simulink model "exjobbtest"  (R2019b)
settings: Solver=VariableStepAuto  StartTime=0.0  StopTime=50  RelTol=1e-3
libraries: simulink x1
settings Model: Creator=Jonathan  LastModifiedBy=Jonathan

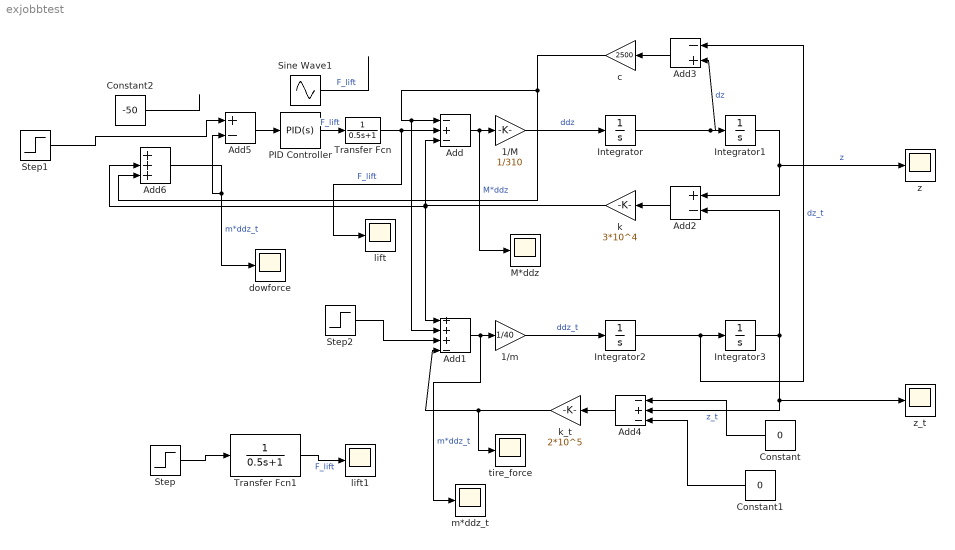
== system exjobbtest ==
  1/M : Gain  Gain=1/310
  1/m : Gain  Gain=1/40
  Add : Sum  Inputs=-+-
  Add1 : Sum  Inputs=+++-
  Add2 : Sum  Inputs=+-
  Add3 : Sum  Inputs=-+
  Add4 : Sum  Inputs=-+-
  Add5 : Sum  Inputs=+-
  Add6 : Sum  Inputs=+++
  Constant : Constant  Value=0
  Constant1 : Constant  Value=0
  Constant2 : Constant  Value=-50
  Integrator{,1..3} (4 alike) : Integrator
  M*ddz : Scope
  PID Controller : simulink/Continuous/PID Controller  Controller=PID  Form=Parallel  TimeDomain=Continuous-time  SampleTime=-1  IntegratorMethod=Forward Euler  FilterMethod=Forward Euler  ControllerParametersSource=internal  P=2.01508415148749  I=5.2932455765264  D=0.107676249350259  UseFilter=on  N=622.23893697959  TunerSelectOption=Transfer Function Based (PID Tuner App)  InitialConditionSource=internal  InitialConditionForIntegrator=0  InitialConditionForFilter=0  DifferentiatorICPrevScaledInput=0  ExternalReset=none  TrackingMode=off  Kt=1  LimitOutput=off  UpperSaturationLimit=inf  LowerSaturationLimit=-inf  LinearizeAsGain=on  AntiWindupMode=none  Kb=1  POutMin=[]  POutMax=[]  IOutMin=[]  IOutMax=[]  DOutMin=[]  DOutMax=[]  NOutMin=[]  NOutMax=[]  SumOutMin=[]  SumOutMax=[]  SaturationOutMin=[]  SaturationOutMax=[]  PParamMin=[]  PParamMax=[]  IParamMin=[]  IParamMax=[]  DParamMin=[]  DParamMax=[]  NParamMin=[]  NParamMax=[]  KbParamMin=[]  KbParamMax=[]  KtParamMin=[]  KtParamMax=[]  KbOutMin=[]  KbOutMax=[]  KtOutMin=[]  KtOutMax=[]  IntegratorOutMin=[]  IntegratorOutMax=[]  FilterOutMin=[]  FilterOutMax=[]  SumI1OutMin=[]  SumI1OutMax=[]  SumI2OutMin=[]  SumI2OutMax=[]  SumI3OutMin=[]  SumI3OutMax=[]  SumI4OutMin=[]  SumI4OutMax=[]  SumDOutMin=[]  SumDOutMax=[]  DifferentiatorOutMin=[]  DifferentiatorOutMax=[]  FilterDiffOutCoefMin=[]  FilterDiffOutCoefMax=[]  ReciprocalOutMin=[]  ReciprocalOutMax=[]  SumDenOutMin=[]  SumDenOutMax=[]  SumNumOutMin=[]  SumNumOutMax=[]  DivideOutMin=[]  DivideOutMax=[]  IntegratorContinuousStateAttributes=''  IntegratorStateMustResolveToSignalObject=off  IntegratorRTWStateStorageClass=Auto  FilterContinuousStateAttributes=''  FilterStateMustResolveToSignalObject=off  FilterRTWStateStorageClass=Auto  ParallelPVariant=InternalParameters  IdealPVariant=Disabled  IVariant=InternalParameters  DVariant=InternalParameters  IntegratorVariant=Continuous  SatVariant=Disabled  AWVariant=Passthrough  PCopyVariant=Disabled  TRVariant=Disabled  FdbkBlocksVariant=Forward  IdealPFdbkVariant=Disabled  SatFdbkVariant=Disabled  DerivativeFilterVariant=ContFilter  NVariant=InternalParameters  NCopyVariant=Disabled  FilterICVariant=InternalICsFilter  IntegratorICVariant=InternalICs  ExternalResetVariant=Disabled  TRSumVariant=Passthrough  SumFdbkVariant=Disabled  SumVariant=Sum_PID
  Sine Wave1 : Sin  SampleTime=0
  Step : Step  Time=0  After=10  SampleTime=0
  Step1 : Step  Time=10  Before=-30  After=-50  SampleTime=0
  Step2 : Step  Time=20  After=20  SampleTime=0
  Transfer Fcn : TransferFcn  Denominator=[0.5 1]
  Transfer Fcn1 : TransferFcn  Denominator=[0.5 1]
  c : Gain  Gain=2500
  dowforce : Scope
  k : Gain  Gain=3*10^4
  "k_t " : Gain  Gain=2*10^5
  lift : Scope
  lift1 : Scope
  m*ddz_t : Scope
  tire_force : Scope
  z : Scope
  z_t : Scope
  wires:
  Integrator/1 -> Add3/2, Integrator1/1  "dz"
  1/M/1 -> Integrator/1  "ddz"
  Integrator1/1 -> z/1, Add2/1  "z"
  k/1 -> Add6/2, Add1/1, Add/3
  1/m/1 -> Integrator2/1  "ddz_t"
  Integrator3/1 -> Add2/2, z_t/1, Add4/2  "z_t"
  Integrator2/1 -> Add3/1, Integrator3/1  "dz_t"
  Add/1 -> M*ddz/1, 1/M/1  "M*ddz"
  Add1/1 -> 1/m/1, m*ddz_t/1  "m*ddz_t"
  Add2/1 -> k/1
  Add3/1 -> c/1
  c/1 -> Add6/3, Add1/2, Add/1
  Add4/1 -> "k_t "/1
  "k_t "/1 -> tire_force/1, Add1/4
  Constant/1 -> Add4/1
  Add5/1 -> PID Controller/1
  Constant1/1 -> Add4/3
  Sine Wave1/1 -> ?  "F_lift"
  Transfer Fcn/1 -> lift/1, Add/2  "F_lift"
  Constant2/1 -> ?
  Add6/1 -> dowforce/1, Add5/2  "m*ddz_t"
  PID Controller/1 -> Transfer Fcn/1  "F_lift"
  Step/1 -> Transfer Fcn1/1
  Transfer Fcn1/1 -> lift1/1  "F_lift"
  Step1/1 -> Add5/1
  Step2/1 -> Add1/3
